simulink model "AMCLIB_SpeedLoop_BAM"  (Simulink 9.3)
settings: Solver=VariableStepAuto  StartTime=0.0  StopTime=10.0  RelTol=1e-3
settings Model: Creator=nxa18952  LastModifiedBy=nxa18952
settings DataIOCC: SaveFormat=Dataset  SignalLoggingSaveFormat=Dataset  ReturnWorkspaceOutputs=on
settings OptimizationCC: LifeSpan=auto
settings DebuggingCC: UnderspecifiedInitializationDetection=Simplified  MergeDetectMultiDrivingBlocksExec=error  FcnCallInpInsideContextMsg=error  SFUnexpectedBacktrackingDiag=error  SFNoUnconditionalDefaultTransitionDiag=error  SFExecutionAtInitializationDiag=warning  ArithmeticOperatorsInVariantConditions=error
settings HardwareCC: ProdBitPerPointer=64  ProdBitPerSizeT=64  ProdBitPerPtrDiffT=64  ProdLargestAtomicFloat=Float  ProdIntDivRoundTo=Zero  ProdEndianess=LittleEndian  ProdWordSize=64  ProdHWDeviceType=Intel->x86-64 (Windows64)
settings ModelReferenceCC: PropagateSignalLabelsOutOfModel=on
settings SFSimCC: SimUseLocalCustomCode=on
settings RTWCC: RTWUseLocalCustomCode=on
settings CodeAppCC: StateflowObjectComments=off
settings GRTTargetCC: TargetLangStandard=C99 (ISO)  CombineOutputUpdateFcns=on  GRTInterface=off
settings ConfigComp: CovMetricSettings=dwe  CovHtmlReporting=off  CovSaveCumulativeToWorkspaceVar=off  CovSaveSingleToWorkspaceVar=off  CovExternalEMLEnable=on

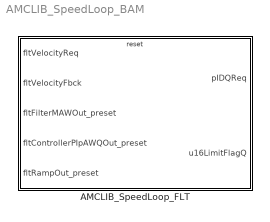
== system AMCLIB_SpeedLoop_BAM ==
  AMCLIB_SpeedLoop_FLT : Subsystem  TreatAsAtomicUnit=on  mask(AMCLIB_SpeedLoop_FLT){showStates=Hide (faster execution), resetStatesEnable=Pre-set according to the first set of inputs after reset, showDebugOutputs=Hide, fltLambdaW=0, fltPropGainQ=0, fltIntegGainQ=0, fltLowerLimitQ=0, fltUpperLimitQ=0, fltRampUp=0, fltRampDown=0}
      mask prompts: showStates "Show internal states"; resetStatesEnable "Internal state after reset"; showDebugOutputs "Show debugging outputs"; fltLambdaW "fltLambdaW (GDFLIB_FilterMA - smoothing factor)"; fltPropGainQ "fltPropGainQ (GFLIB_ControllerPIpAW - proportional gain)"; fltIntegGainQ "fltIntegGainQ (GFLIB_ControllerPIpAW - integral gain)"; fltLowerLimitQ "fltLowerLimitQ (GFLIB_ControllerPIpAW - lower limit)"; fltUpperLimitQ "fltUpperLimitQ (GFLIB_ControllerPIpAW - upper limit)"; fltRampUp "fltRampUp (Ramp up increment coefficient)"; fltRampDown "fltRampDown (Ramp decrement coefficient)"
      mask help: Speed loop controller for the PMSM field-oriented control algorithm in single precision floating-point implementation. This block supports re-initialization of the internal state during simulation. If the block is reset, the outputs of the MA filter, PI controller, and the ramp will be aligned with the inputs fltFilterMAWOut_preset, fltControllerPIpAWQOut_preset, and fltRampOut_preset. Refer to the AMMCLIB User's Guide for further details.
      mask init:
      | if ~evalin('base','exist(''tS8'',''var'')')
      |   if (2 ~= exist('SWLIBS_Typedefs.mat','file'))
      |       error('File SWLIBS_Typedefs.mat is not on the Matlab path. Please add the AMMCLIB "bam" folder in the Matlab Search Path.');
      |   else
      |       evalin('base', 'load(''SWLIBS_Typedefs.mat'')');
      |   end
      | end
      | if showStates == 1
      |     % hidden state variables
      |     if strcmp(get_param([gcb '/fltLambdaW'], 'BlockType'), 'Inport')
      |         posblk = get_param(gcb, 'Position');
      | 
      |         pos = get_param(    [gcb, '/fltLambdaW'], 'Position');
      |         orient = get_param( [gcb, '/fltLambdaW'], 'Orientation');
      |         delete_block(       [gcb, '/fltLambdaW']);
      |         add_block('built-in/Ground', [gcb, '/fltLambdaW'], 'Position', pos, 'Orientation', orient);
      | 
      |         pos = get_param(    [gcb, '/fltPropGainQ'], 'Position');
      |         orient = get_param( [gcb, '/fltPropGainQ'], 'Orientation');
      |         delete_block(       [gcb, '/fltPropGainQ']);
      |         add_block('built-in/Ground', [gcb, '/fltPropGainQ'], 'Position', pos, 'Orientation', orient);
      | 
      |         pos = get_param(    [gcb, '/fltIntegGainQ'], 'Position');
      |         orient = get_param( [gcb, '/fltIntegGainQ'], 'Orientation');
      |         delete_block(       [gcb, '/fltIntegGainQ']);
      |         add_block('built-in/Ground', [gcb, '/fltIntegGainQ'], 'Position', pos, 'Orientation', orient);
      | 
      |         pos = get_param(    [gcb, '/fltLowerLimitQ'], 'Position');
      |         orient = get_param( [gcb, '/fltLowerLimitQ'], 'Orientation');
      |         delete_block(       [gcb, '/fltLowerLimitQ']);
      |         add_block('built-in/Ground', [gcb, '/fltLowerLimitQ'], 'Position', pos, 'Orientation', orient);
      | 
      |         pos = get_param(    [gcb, '/fltUpperLimitQ'], 'Position');
      |         orient = get_param( [gcb, '/fltUpperLimitQ'], 'Orientation');
      |         delete_block(       [gcb, '/fltUpperLimitQ']);
      |         add_block('built-in/Ground', [gcb, '/fltUpperLimitQ'], 'Position', pos, 'Orientation', orient);
      | 
      |         pos = get_param(    [gcb, '/fltRampUp'], 'Position');
      |         orient = get_param( [gcb, '/fltRampUp'], 'Orientation');
      |         delete_block(       [gcb, '/fltRampUp']);
      |         add_block('built-in/Ground', [gcb, '/fltRampUp'], 'Position', pos, 'Orientation', orient);
      | 
      |         pos = get_param(    [gcb, '/fltRampDown'], 'Position');
      |         orient = get_param( [gcb, '/fltRampDown'], 'Orientation');
      |         delete_block(       [gcb, '/fltRampDown']);
      |         add_block('built-in/Ground', [gcb, '/fltRampDown'], 'Position', pos, 'Orientation', orient);
      | 
      |         pos = get_param(    [gcb, '/fltAccW'], 'Position');
      |         orient = get_param( [gcb, '/fltAccW'], 'Orientation');
      |         delete_block(       [gcb, '/fltAccW']);
      |         add_block('built-in/Ground', [gcb, '/fltAccW'], 'Position', pos, 'Orientation', orient);
      | 
      |         pos = get_param(    [gcb, '/fltIntegPartK_1Q'], 'Position');
      |         orient = get_param( [gcb, '/fltIntegPartK_1Q'], 'Orientation');
      |         delete_block(       [gcb, '/fltIntegPartK_1Q']);
      |         add_block('built-in/Ground', [gcb, '/fltIntegPartK_1Q'], 'Position', pos, 'Orientation', orient);
      | 
      |         pos = get_param(    [gcb, '/fltInK_1Q'], 'Position');
      |         orient = get_param( [gcb, '/fltInK_1Q'], 'Orientation');
      |         delete_block(       [gcb, '/fltInK_1Q']);
      |         add_block('built-in/Ground', [gcb, '/fltInK_1Q'], 'Position', pos, 'Orientation', orient);
      | 
      |         pos = get_param(    [gcb, '/fltState'], 'Position');
      |         orient = get_param( [gcb, '/fltState'], 'Orientation');
      |         delete_block(       [gcb, '/fltState']);
      |         add_block('built-in/Ground', [gcb, '/fltState'], 'Position', pos, 'Orientation', orient);
      | 
      | 
      |         pos = get_param(    [gcb '/fltAccW_Out'], 'Position');
      |         orient = get_param( [gcb '/fltAccW_Out'], 'Orientation');
      |         delete_block(       [gcb '/fltAccW_Out']);
      |         add_block('built-in/Terminator', [gcb '/fltAccW_Out'], 'Position', pos, 'Orientation', orient);
      | 
      |         pos = get_param(    [gcb '/fltIntegPartK_1Q_Out'], 'Position');
      |         orient = get_param( [gcb '/fltIntegPartK_1Q_Out'], 'Orientation');
      |         delete_block(       [gcb '/fltIntegPartK_1Q_Out']);
      |         add_block('built-in/Terminator', [gcb '/fltIntegPartK_1Q_Out'], 'Position', pos, 'Orientation', orient);
      | 
      |         pos = get_param(    [gcb '/fltInK_1Q_Out'], 'Position');
      |         orient = get_param( [gcb '/fltInK_1Q_Out'], 'Orientation');
      |         delete_block(       [gcb '/fltInK_1Q_Out']);
      |         add_block('built-in/Terminator', [gcb '/fltInK_1Q_Out'], 'Position', pos, 'Orientation', orient);
      | 
      |         pos = get_param(    [gcb '/fltState_Out'], 'Position');
      |         orient = get_param( [gcb '/fltState_Out'], 'Orientation');
      |         delete_block(       [gcb '/fltState_Out']);
      |         add_block('built-in/Terminator', [gcb '/fltState_Out'], 'Position', pos, 'Orientation', orient);
      | 
      | 
      |         if strcmp(get_param([gcb '/fltWReqFilt'], 'BlockType'), 'Outport')
      |             pos = get_param(    [gcb '/fltWReqFilt'], 'Position');
      |             orient = get_param( [gcb '/fltWReqFilt'], 'Orientation');
      |             delete_block(       [gcb '/fltWReqFilt']);
      |             add_block('built-in/Terminator', [gcb '/fltWReqFilt'], 'Position', pos, 'Orientation', orient);
      | 
      |             pos = get_param(    [gcb '/fltWErr'], 'Position');
      |             orient = get_param( [gcb '/fltWErr'], 'Orientation');
      |             delete_block(       [gcb '/fltWErr']);
      |             add_block('built-in/Terminator', [gcb '/fltWErr'], 'Position', pos, 'Orientation', orient);
      | 
      |             pos = get_param(    [gcb '/fltWFbckFilt'], 'Position');
      |             orient = get_param( [gcb '/fltWFbckFilt'], 'Orientation');
      |             delete_block(       [gcb '/fltWFbckFilt']);
      |             add_block('built-in/Terminator', [gcb '/fltWFbckFilt'], 'Position', pos, 'Orientation', orient);
      | 
      |         end
      | 
      |         set_param([gcb '/fltVelocityReq'], 'Port', '1');
      |         set_param([gcb '/fltVelocityFbck'], 'Port', '2');
      |         set_param([gcb '/fltFilterMAWOut_preset'], 'Port', '3');
      |         set_param([gcb '/fltControllerPIpAWQOut_preset'], 'Port', '4');
      |         set_param([gcb '/fltRampOut_preset'], 'Port', '5');
      | 
      |         set_param([gcb '/pIDQReq'], 'Port', '1');
      |         set_param([gcb '/u16LimitFlagQ'], 'Port', '2');
      | 
      |         set_param(gcb,'MaskEnables',{'on','on','off','on','on','on','on','on','on','on'});
      | 
      |         if (posblk(4) - posblk(2)) > 150
      |           height = 150;
      |           set_param(gcb,'Position',[posblk(1), posblk(2), posblk(3), posblk(2)+height])
      |         end
      |     end
      | else
      |     % shown state variables
      |     if strcmp(get_param([gcb '/fltLambdaW'], 'BlockType'), 'Ground')
      |         posblk = get_param(gcb, 'Position');
      | 
      |         pos = get_param(    [gcb, '/fltLambdaW'], 'Position');
      |         orient = get_param( [gcb, '/fltLambdaW'], 'Orientation');
      |         delete_block(       [gcb, '/fltLambdaW']);
      |         add_block('built-in/Inport', [gcb, '/fltLambdaW'], 'Position', pos, 'Orientation', orient, 'OutDataTypeStr', 'single');
      | 
      |         pos = get_param(    [gcb, '/fltPropGainQ'], 'Position');
      |         orient = get_param( [gcb, '/fltPropGainQ'], 'Orientation');
      |         delete_block(       [gcb, '/fltPropGainQ']);
      |         add_block('built-in/Inport', [gcb, '/fltPropGainQ'], 'Position', pos, 'Orientation', orient, 'OutDataTypeStr', 'single');
      | 
      |         pos = get_param(    [gcb, '/fltIntegGainQ'], 'Position');
      |         orient = get_param( [gcb, '/fltIntegGainQ'], 'Orientation');
      |         delete_block(       [gcb, '/fltIntegGainQ']);
      |         add_block('built-in/Inport', [gcb, '/fltIntegGainQ'], 'Position', pos, 'Orientation', orient, 'OutDataTypeStr', 'single');
      | 
      |         pos = get_param(    [gcb, '/fltLowerLimitQ'], 'Position');
      |         orient = get_param( [gcb, '/fltLowerLimitQ'], 'Orientation');
      |         delete_block(       [gcb, '/fltLowerLimitQ']);
      |         add_block('built-in/Inport', [gcb, '/fltLowerLimitQ'], 'Position', pos, 'Orientation', orient, 'OutDataTypeStr', 'single');
      | 
      |         pos = get_param(    [gcb, '/fltUpperLimitQ'], 'Position');
      |         orient = get_param( [gcb, '/fltUpperLimitQ'], 'Orientation');
      |         delete_block(       [gcb, '/fltUpperLimitQ']);
      |         add_block('built-in/Inport', [gcb, '/fltUpperLimitQ'], 'Position', pos, 'Orientation', orient, 'OutDataTypeStr', 'single');
      | 
      |         pos = get_param(    [gcb, '/fltRampUp'], 'Position');
      |         orient = get_param( [gcb, '/fltRampUp'], 'Orientation');
      |         delete_block(       [gcb, '/fltRampUp']);
      |         add_block('built-in/Inport', [gcb, '/fltRampUp'], 'Position', pos, 'Orientation', orient, 'OutDataTypeStr', 'single');
      | 
      |         pos = get_param(    [gcb, '/fltRampDown'], 'Position');
      |         orient = get_param( [gcb, '/fltRampDown'], 'Orientation');
      |         delete_block(       [gcb, '/fltRampDown']);
      |         add_block('built-in/Inport', [gcb, '/fltRampDown'], 'Position', pos, 'Orientation', orient, 'OutDataTypeStr', 'single');
      | 
      |         pos = get_param(    [gcb, '/fltAccW'], 'Position');
      |         orient = get_param( [gcb, '/fltAccW'], 'Orientation');
      |         delete_block(       [gcb, '/fltAccW']);
      |         add_block('built-in/Inport', [gcb, '/fltAccW'], 'Position', pos, 'Orientation', orient, 'OutDataTypeStr', 'single');
      | 
      |         pos = get_param(    [gcb, '/fltIntegPartK_1Q'], 'Position');
      |         orient = get_param( [gcb, '/fltIntegPartK_1Q'], 'Orientation');
      |         delete_block(       [gcb, '/fltIntegPartK_1Q']);
      |         add_block('built-in/Inport', [gcb, '/fltIntegPartK_1Q'], 'Position', pos, 'Orientation', orient, 'OutDataTypeStr', 'single');
      | 
      |         pos = get_param(    [gcb, '/fltInK_1Q'], 'Position');
      |         orient = get_param( [gcb, '/fltInK_1Q'], 'Orientation');
      |         delete_block(       [gcb, '/fltInK_1Q']);
      |         add_block('built-in/Inport', [gcb, '/fltInK_1Q'], 'Position', pos, 'Orientation', orient, 'OutDataTypeStr', 'single');
      | 
      |         pos = get_param(    [gcb, '/fltState'], 'Position');
      |         orient = get_param( [gcb, '/fltState'], 'Orientation');
      |         delete_block(       [gcb, '/fltState']);
      |         add_block('built-in/Inport', [gcb, '/fltState'], 'Position', pos, 'Orientation', orient, 'OutDataTypeStr', 'single');
      | 
      | 
      |         pos = get_param(    [gcb '/fltAccW_Out'], 'Position');
      |         orient = get_param( [gcb '/fltAccW_Out'], 'Orientation');
      |         delete_block(       [gcb '/fltAccW_Out']);
      |         add_block('built-in/Outport', [gcb '/fltAccW_Out'], 'Position', pos, 'Orientation', orient);
      | 
      |         pos = get_param(    [gcb '/fltIntegPartK_1Q_Out'], 'Position');
      |         orient = get_param( [gcb '/fltIntegPartK_1Q_Out'], 'Orientation');
      |         delete_block(       [gcb '/fltIntegPartK_1Q_Out']);
      |         add_block('built-in/Outport', [gcb '/fltIntegPartK_1Q_Out'], 'Position', pos, 'Orientation', orient);
      | 
      |         pos = get_param(    [gcb '/fltInK_1Q_Out'], 'Position');
      |         orient = get_param( [gcb '/fltInK_1Q_Out'], 'Orientation');
      |         delete_block(       [gcb '/fltInK_1Q_Out']);
      |         add_block('built-in/Outport', [gcb '/fltInK_1Q_Out'], 'Position', pos, 'Orientation', orient);
      | 
      |         pos = get_param(    [gcb '/fltState_Out'], 'Position');
      |         orient = get_param( [gcb '/fltState_Out'], 'Orientation');
      |         delete_block(       [gcb '/fltState_Out']);
      |         add_block('built-in/Outport', [gcb '/fltState_Out'], 'Position', pos, 'Orientation', orient);
      | 
      | 
      |         if (showDebugOutputs == 2) && (strcmp(get_param([gcb '/fltWReqFilt'], 'BlockType'), 'Terminator'))
      |             pos = get_param(    [gcb '/fltWReqFilt'], 'Position');
      |             orient = get_param( [gcb '/fltWReqFilt'], 'Orientation');
      |             delete_block(       [gcb '/fltWReqFilt']);
      |             add_block('built-in/Outport', [gcb '/fltWReqFilt'], 'Position', pos, 'Orientation', orient);
      | 
      |             pos = get_param(    [gcb '/fltWErr'], 'Position');
      |             orient = get_param( [gcb '/fltWErr'], 'Orientation');
      |             delete_block(       [gcb '/fltWErr']);
      |             add_block('built-in/Outport', [gcb '/fltWErr'], 'Position', pos, 'Orientation', orient);
      | 
      |             pos = get_param(    [gcb '/fltWFbckFilt'], 'Position');
      |             orient = get_param( [gcb '/fltWFbckFilt'], 'Orientation');
      |             delete_block(       [gcb '/fltWFbckFilt']);
      |             add_block('built-in/Outport', [gcb '/fltWFbckFilt'], 'Position', pos, 'Orientation', orient);
      | 
      |         end
      | 
      |         set_param([gcb '/fltVelocityReq'], 'Port', '1');
      |         set_param([gcb '/fltVelocityFbck'], 'Port', '2');
      |         set_param([gcb '/fltFilterMAWOut_preset'], 'Port', '3');
      |         set_param([gcb '/fltControllerPIpAWQOut_preset'], 'Port', '4');
      |         set_param([gcb '/fltRampOut_preset'], 'Port', '5');
      |         set_param([gcb '/fltLambdaW'], 'Port', '6');
      |         set_param([gcb '/fltPropGainQ'], 'Port', '7');
      |         set_param([gcb '/fltIntegGainQ'], 'Port', '8');
      |         set_param([gcb '/fltLowerLimitQ'], 'Port', '9');
      |         set_param([gcb '/fltUpperLimitQ'], 'Port', '10');
      |         set_param([gcb '/fltRampUp'], 'Port', '11');
      |         set_param([gcb '/fltRampDown'], 'Port', '12');
      |         set_param([gcb '/fltAccW'], 'Port', '13');
      |         set_param([gcb '/fltIntegPartK_1Q'], 'Port', '14');
      |         set_param([gcb '/fltInK_1Q'], 'Port', '15');
      |         set_param([gcb '/fltState'], 'Port', '16');
      | 
      |         if (showDebugOutputs == 2)
      |             set_param([gcb '/pIDQReq'], 'Port', '1');
      |             set_param([gcb '/u16LimitFlagQ'], 'Port', '2');
      |             set_param([gcb '/fltWReqFilt'], 'Port', '3');
      |             set_param([gcb '/fltWErr'], 'Port', '4');
      |             set_param([gcb '/fltWFbckFilt'], 'Port', '5');
      |             set_param([gcb '/fltAccW_Out'], 'Port', '6');
      |             set_param([gcb '/fltIntegPartK_1Q_Out'], 'Port', '7');
      |             set_param([gcb '/fltInK_1Q_Out'], 'Port', '8');
      |             set_param([gcb '/fltState_Out'], 'Port', '9');
      |         else
      |             set_param([gcb '/pIDQReq'], 'Port', '1');
      |             set_param([gcb '/u16LimitFlagQ'], 'Port', '2');
      |             set_param([gcb '/fltAccW_Out'], 'Port', '3');
      |             set_param([gcb '/fltIntegPartK_1Q_Out'], 'Port', '4');
      |             set_param([gcb '/fltInK_1Q_Out'], 'Port', '5');
      |             set_param([gcb '/fltState_Out'], 'Port', '6');
      |         end
      | 
      |         set_param(gcb,'MaskEnables',{'on','on','on','off','off','off','off','off','off','off'});
      | 
      |         if (posblk(4) - posblk(2)) < 425
      |           height = 425;
      |           set_param(gcb,'Position',[posblk(1), posblk(2), posblk(3), posblk(2)+height])
      |         end
      |     else
      |         if (showDebugOutputs == 2) && (strcmp(get_param([gcb '/fltWReqFilt'], 'BlockType'), 'Terminator'))
      |             % shown debugging outputs
      |             pos = get_param(    [gcb '/fltWReqFilt'], 'Position');
      |             orient = get_param( [gcb '/fltWReqFilt'], 'Orientation');
      |             delete_block(       [gcb '/fltWReqFilt']);
      |             add_block('built-in/Outport', [gcb '/fltWReqFilt'], 'Position', pos, 'Orientation', orient);
      | 
      |             pos = get_param(    [gcb '/fltWErr'], 'Position');
      |             orient = get_param( [gcb '/fltWErr'], 'Orientation');
      |             delete_block(       [gcb '/fltWErr']);
      |             add_block('built-in/Outport', [gcb '/fltWErr'], 'Position', pos, 'Orientation', orient);
      | 
      |             pos = get_param(    [gcb '/fltWFbckFilt'], 'Position');
      |             orient = get_param( [gcb '/fltWFbckFilt'], 'Orientation');
      |             delete_block(       [gcb '/fltWFbckFilt']);
      |             add_block('built-in/Outport', [gcb '/fltWFbckFilt'], 'Position', pos, 'Orientation', orient);
      | 
      |             set_param([gcb '/pIDQReq'], 'Port', '1');
      |             set_param([gcb '/u16LimitFlagQ'], 'Port', '2');
      |             set_param([gcb '/fltWReqFilt'], 'Port', '3');
      |             set_param([gcb '/fltWErr'], 'Port', '4');
      |             set_param([gcb '/fltWFbckFilt'], 'Port', '5');
      |             set_param([gcb '/fltAccW_Out'], 'Port', '6');
      |             set_param([gcb '/fltIntegPartK_1Q_Out'], 'Port', '7');
      |             set_param([gcb '/fltInK_1Q_Out'], 'Port', '8');
      |             set_param([gcb '/fltState_Out'], 'Port', '9');
      |         elseif (showDebugOutputs == 1) && (strcmp(get_param([gcb '/fltWReqFilt'], 'BlockType'), 'Outport'))
      |             % hidden debugging outputs
      |             pos = get_param(    [gcb '/fltWReqFilt'], 'Position');
      |             orient = get_param( [gcb '/fltWReqFilt'], 'Orientation');
      |             delete_block(       [gcb '/fltWReqFilt']);
      |             add_block('built-in/Terminator', [gcb '/fltWReqFilt'], 'Position', pos, 'Orientation', orient);
      | 
      |             pos = get_param(    [gcb '/fltWErr'], 'Position');
      |             orient = get_param( [gcb '/fltWErr'], 'Orientation');
      |             delete_block(       [gcb '/fltWErr']);
      |             add_block('built-in/Terminator', [gcb '/fltWErr'], 'Position', pos, 'Orientation', orient);
      | 
      |             pos = get_param(    [gcb '/fltWFbckFilt'], 'Position');
      |             orient = get_param( [gcb '/fltWFbckFilt'], 'Orientation');
      |             delete_block(       [gcb '/fltWFbckFilt']);
      |             add_block('built-in/Terminator', [gcb '/fltWFbckFilt'], 'Position', pos, 'Orientation', orient);
      | 
      |             set_param([gcb '/pIDQReq'], 'Port', '1');
      |             set_param([gcb '/u16LimitFlagQ'], 'Port', '2');
      |             set_param([gcb '/fltAccW_Out'], 'Port', '3');
      |             set_param([gcb '/fltIntegPartK_1Q_Out'], 'Port', '4');
      |             set_param([gcb '/fltInK_1Q_Out'], 'Port', '5');
      |             set_param([gcb '/fltState_Out'], 'Port', '6');
      |         end
      |     end
      | end
      settings: RTWSystemCode=Inline
      mask TypeOptions showStates: Hide (faster execution) | Show (allows debugging; connect feedback loops manually)
      mask Callback showStates:
      | maskStr = get_param(gcb,'showStates');
      | if strcmp(maskStr,'Hide (faster execution)'),
      |     set_param(gcb,'MaskEnables',{'on','on','off','on','on','on','on','on','on','on'});
      | else
      |     set_param(gcb,'MaskEnables',{'on','on','on','off','off','off','off','off','off','off'});
      | end
      mask TypeOptions resetStatesEnable: Pre-set according to the first set of inputs after reset | Clear to zero
      mask TypeOptions showDebugOutputs: Hide | Show
      mask Display:
      | color('black');
      | pos = get_param(gcb, 'Position');
      | width = pos(3) - pos(1);
      | height = pos(4) - pos(2);
      | tX=width/2;
      | tY=height - 25;
      | color('black');
      | text(tX,tY, 'AMCLIB_SpeedLoop_FLT', 'horizontalAlignment', 'center');
      | if showStates == 2
      |   color('red');
      |   text(tX,tY - 20, ['debugging mode' char(13) char(10) '(limited performance)'], 'horizontalAlignment', 'center');
      | end

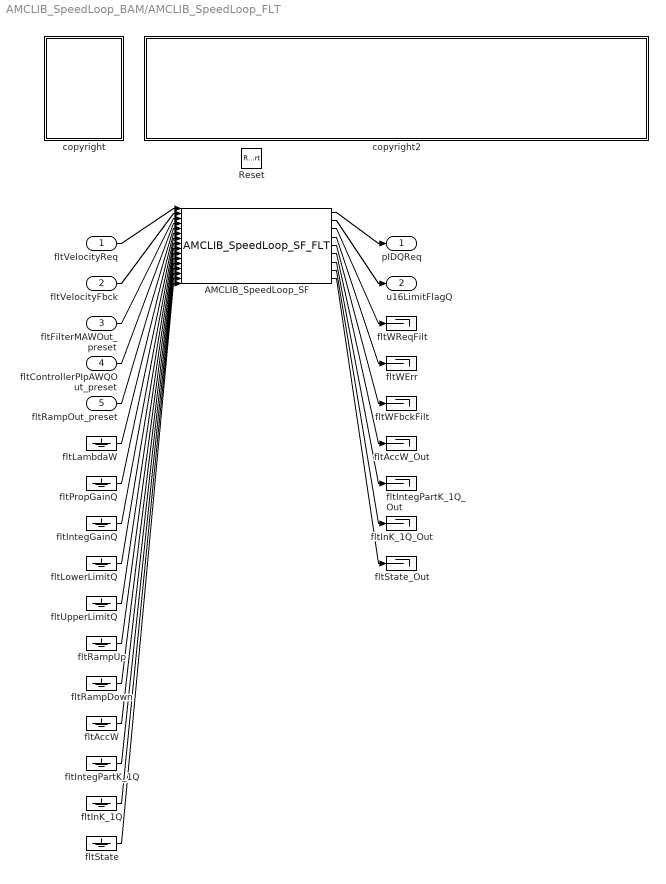
== system AMCLIB_SpeedLoop_BAM/AMCLIB_SpeedLoop_FLT ==
  fltVelocityReq : Inport  OutDataTypeStr=single
  fltVelocityFbck : Inport  Port=2  OutDataTypeStr=single
  fltFilterMAWOut_preset : Inport  Port=3  OutDataTypeStr=single
  fltControllerPIpAWQOut_preset : Inport  Port=4  OutDataTypeStr=single
  fltRampOut_preset : Inport  Port=5  OutDataTypeStr=single
  Reset : ResetPort  DisableCoverage=on
  AMCLIB_SpeedLoop_SF : S-Function  FunctionName=AMCLIB_SpeedLoop_SF_FLT  Parameters=showStates,resetStatesEnable,showDebugOutputs,fltLambdaW,fltPropGainQ,fltIntegGainQ,fltLowerLimitQ,fltUpperLimitQ,fltRampUp,fltRampDown  SFunctionDeploymentMode=off  EnableBusSupport=off
  copyright : Subsystem
      mask Display: text(10,90,'FILE:');text(10,75,'DESRIPTION:');text(10,60,'COPYRIGHT:');text(10,45,'VERSION:');text(10,30,'DATE:')
  copyright2 : Subsystem
      mask Display: text(10,90,'AMCLIB_SpeedLoop_BAM_FLT.mdl');text(10,75,'PMSM Speed Loop Controller.');text(10,60,'NXP 2020');text(10,45,'1.0');text(10,30,'28-Mar-2020');
  fltAccW : Ground
  fltAccW_Out : Terminator
  fltInK_1Q : Ground
  fltInK_1Q_Out : Terminator
  fltIntegGainQ : Ground
  fltIntegPartK_1Q : Ground
  fltIntegPartK_1Q_Out : Terminator
  fltLambdaW : Ground
  fltLowerLimitQ : Ground
  fltPropGainQ : Ground
  fltRampDown : Ground
  fltRampUp : Ground
  fltState : Ground
  fltState_Out : Terminator
  fltUpperLimitQ : Ground
  fltWErr : Terminator
  fltWFbckFilt : Terminator
  fltWReqFilt : Terminator
  pIDQReq : Outport
  u16LimitFlagQ : Outport  Port=2
  wires:
  fltVelocityReq/1 -> AMCLIB_SpeedLoop_SF/1
  fltVelocityFbck/1 -> AMCLIB_SpeedLoop_SF/2
  fltFilterMAWOut_preset/1 -> AMCLIB_SpeedLoop_SF/3
  fltControllerPIpAWQOut_preset/1 -> AMCLIB_SpeedLoop_SF/4
  fltRampOut_preset/1 -> AMCLIB_SpeedLoop_SF/5
  fltLambdaW/1 -> AMCLIB_SpeedLoop_SF/6
  fltPropGainQ/1 -> AMCLIB_SpeedLoop_SF/7
  fltIntegGainQ/1 -> AMCLIB_SpeedLoop_SF/8
  fltLowerLimitQ/1 -> AMCLIB_SpeedLoop_SF/9
  fltUpperLimitQ/1 -> AMCLIB_SpeedLoop_SF/10
  fltRampUp/1 -> AMCLIB_SpeedLoop_SF/11
  fltRampDown/1 -> AMCLIB_SpeedLoop_SF/12
  fltAccW/1 -> AMCLIB_SpeedLoop_SF/13
  fltIntegPartK_1Q/1 -> AMCLIB_SpeedLoop_SF/14
  fltInK_1Q/1 -> AMCLIB_SpeedLoop_SF/15
  fltState/1 -> AMCLIB_SpeedLoop_SF/16
  AMCLIB_SpeedLoop_SF/1 -> pIDQReq/1
  AMCLIB_SpeedLoop_SF/2 -> u16LimitFlagQ/1
  AMCLIB_SpeedLoop_SF/3 -> fltWReqFilt/1
  AMCLIB_SpeedLoop_SF/4 -> fltWErr/1
  AMCLIB_SpeedLoop_SF/5 -> fltWFbckFilt/1
  AMCLIB_SpeedLoop_SF/6 -> fltAccW_Out/1
  AMCLIB_SpeedLoop_SF/7 -> fltIntegPartK_1Q_Out/1
  AMCLIB_SpeedLoop_SF/8 -> fltInK_1Q_Out/1
  AMCLIB_SpeedLoop_SF/9 -> fltState_Out/1

== system AMCLIB_SpeedLoop_BAM/AMCLIB_SpeedLoop_FLT/copyright ==

== system AMCLIB_SpeedLoop_BAM/AMCLIB_SpeedLoop_FLT/copyright2 ==
